simulink model "move_to_pose_R2020a"  (R2020b)
settings: Solver=FixedStepAuto  StartTime=0.0  StopTime=inf  FixedStep=sampleTime  RelTol=1e-3
PreLoadFcn:
  | % Simulation parameters
  | load exampleMap
  | sampleTime = 0.05;
  | 
  | % Robot parameters
  | wheelRadius = 0.05;
  | robotRadius = 0.5;
  | 
  | % Lidar parameters
  | sensorOffset = [0,0];
  | scanAngles = linspace(-pi/2,pi/2,9)';
  | maxRange = 25;
values from neighbouring files (symbols this model uses):
  start = [5,17.5]    [mapgen.m]    (also in path_gen.m = [pose(1) pose(2)])
libraries: mobileRoboticsLib x4, robotalgslib x1, mobileRoboticsTrainingLib x1
settings Model: SimulationMode=accelerator  EnablePacing=on  PacingRate=1000  Creator=scastro  LastModifiedBy=jayas
settings DataIOCC: ReturnWorkspaceOutputs=off
settings DebuggingCC: PregeneratedLibrarySubsystemCodeDiagnostic=none  ArithmeticOperatorsInVariantConditions=warning
settings SFSimCC: SimUseLocalCustomCode=off  CustomCodeUndefinedFunction=UseInterfaceOnly
settings RTWCC: RTWUseLocalCustomCode=off

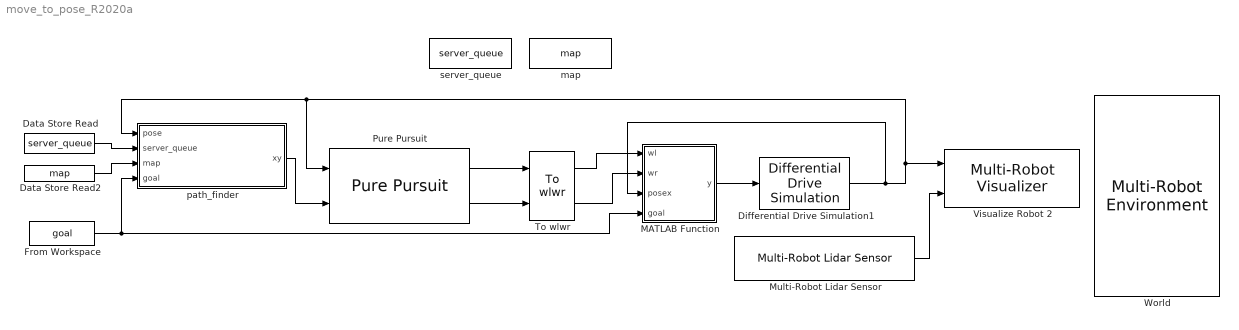
== system move_to_pose_R2020a ==
  Data Store Read : DataStoreRead  DataStoreName=server_queue
  Data Store Read2 : DataStoreRead  DataStoreName=map
  Differential Drive Simulation1 : mobileRoboticsLib/Kinematic Models/Differential Drive/Differential Drive Simulation  wheelRadius=wheelRadius  wheelBase=robotRadius  initX=start(1)  initY=start(2)  initAngle=0  Ts=sampleTime
      settings: SourceProductName=Mobile Robotics Simulation Toolbox
  From Workspace : FromWorkspace  VariableName=goal  SampleTime=-1
  MATLAB Function : MATLAB Function  TreatAsAtomicUnit=on
  Multi-Robot Lidar Sensor : mobileRoboticsLib/Environments/Multi-Robot Lidar Sensor  robotIdx=1  mapName=map  sensorOffset=sensorOffset  scanAngles=scanAngles  maxRange=maxRange
      settings: SourceProductName=Mobile Robotics Simulation Toolbox
  Pure Pursuit : robotalgslib/Pure Pursuit  DesiredLinearVelocity=0.1  MaxAngularVelocity=1  LookaheadDistance=1  TargetDirPort=off  SimulateUsing=Code generation
  To wlwr : mobileRoboticsTrainingLib/To wlwr  axleLength=0.1  wheelR=0.05
  Visualize Robot 2 : mobileRoboticsLib/Environments/Multi-Robot Visualizer  idx=1  radius=robotRadius  robotColor=[1 0 0]  showTraj=off  hasLidar=on  sensorOffset=sensorOffset  scanAngles=scanAngles  maxNumScans=0  hasObjDetector=off  objDetectorOffset=[0,0]  objDetectorAngle=0  objDetectorFOV=pi/2  objDetectorMaxRange=5  hasRobotDetector=off  robotDetectorOffset=sensorOffset  robotDetectorAngle=[pi/2 -pi/2]  robotDetectorFOV=pi  robotDetectorMaxRange=25  robotDetectorNumDetections=0
      link override Goto_ObjDetector: GotoTag=slMultiRobotEnv_ObjDet_2
      link override Goto_RobotDetector: GotoTag=slMultiRobotEnv_RobotDet_2
      settings: SourceProductName=Mobile Robotics Simulation Toolbox
  World : mobileRoboticsLib/Environments/Multi-Robot Environment  numRobots=1  mapName=map  showWaypoints=off  showObjects=off  objectColors=[1 0 0;0 1 0;0 0 1]  objectMarkers='s'  showRobotIds=on  plotSensorLines=on
      settings: SourceProductName=Mobile Robotics Simulation Toolbox
  map : DataStoreMemory  DataStoreName=map  ReadBeforeWriteMsg=warning  WriteAfterWriteMsg=warning  WriteAfterReadMsg=warning  ShowAdditionalParam=off
  path_finder : MATLAB Function  TreatAsAtomicUnit=on
  server_queue : DataStoreMemory  DataStoreName=server_queue  ReadBeforeWriteMsg=warning  WriteAfterWriteMsg=warning  WriteAfterReadMsg=warning  ShowAdditionalParam=off
  wires:
  Multi-Robot Lidar Sensor/1 -> Visualize Robot 2/2
  Pure Pursuit/2 -> To wlwr/2
  Pure Pursuit/1 -> To wlwr/1
  To wlwr/1 -> MATLAB Function/1(wl)
  To wlwr/2 -> MATLAB Function/2(wr)
  MATLAB Function/1(y) -> Differential Drive Simulation1/1
  Differential Drive Simulation1/1 -> MATLAB Function/3(posex), path_finder/1(pose), Pure Pursuit/1, Visualize Robot 2/1
  path_finder/1(xy) -> Pure Pursuit/2
  Data Store Read/1 -> path_finder/2(server_queue)
  Data Store Read2/1 -> path_finder/3(map)
  From Workspace/1 -> MATLAB Function/4(goal), path_finder/4(goal)

== matlab function move_to_pose_R2020a/path_finder ==
  data: xy output; pose input; server_queue input; map input; goal input
function xy = path_finder(pose, server_queue, map, goal)
    xy = path_gen(pose, server_queue, map, goal);
end

== matlab function move_to_pose_R2020a/MATLAB Function ==
  data: wl input; y output; wr input; posex input; goal input
function y = fcn(wl, wr, posex, goal)
%     if (abs(posex(1) - goal(1)) < 0.02 && abs(posex(2) - goal(2)) < 0.02)
%         y = [0 0];
%     else
%         y = [wl, wr];
%     end
    goal
    y = [1 1];
end
